simulink model "Mechanical_sol"  (R2018b)
settings: Solver=VariableStepAuto  StartTime=0.0  StopTime=60  RelTol=1e-3
values from neighbouring files (symbols this model uses):
  Dm = 0.0071    [QuanserData.m]
  Dp = 0.0071    [QuanserData.m]
  Dt = 0.158    [QuanserData.m]
  g = 9.81    [QuanserData.m]
  Jeq = Jm+Jh+Jp    (= 1.120304e-05)    [QuanserData.m]
  Jp = 2.15e-2    (= 0.0215)    [QuanserData.m]
  k1 = 1.2e-5    (= 1.2e-05)    [QuanserData.m]
  k2 = 3.54e-9    (= 3.54e-09)    [QuanserData.m]
  k3 = 0    [QuanserData.m]
  k4 = 6.23e-7    (= 6.23e-07)    [QuanserData.m]
  km = 0.042    [QuanserData.m]
  Lm = 1.16e-3    (= 0.00116)    [QuanserData.m]
  Mb = 1.15    [QuanserData.m]
  Rm = 8.4    [QuanserData.m]
settings Model: Creator=y.briere  LastModifiedBy=y.briere
settings DataIOCC: InitialState=[]  LoadInitialState=on

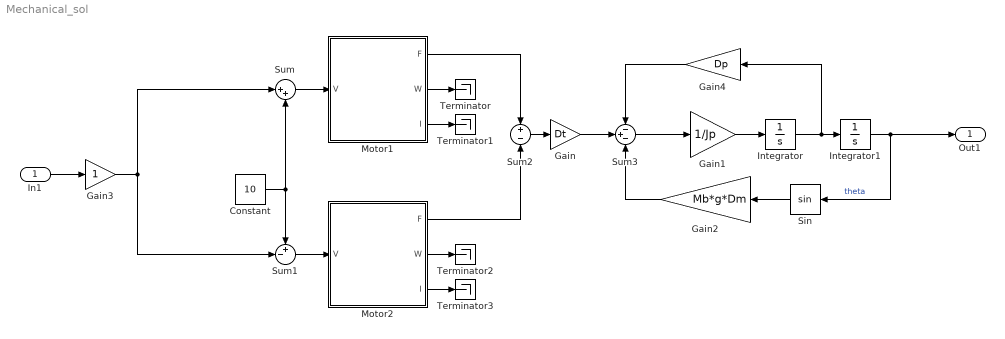
== system Mechanical_sol ==
  In1 : Inport
  Constant : Constant  Value=10
  Gain : Gain  Gain=Dt
  Gain1 : Gain  Gain=1/Jp
  Gain2 : Gain  Gain=Mb*g*Dm
  Gain3 : Gain
  Gain4 : Gain  Gain=Dp
  Integrator : Integrator
  Integrator1 : Integrator
  Motor1 : Subsystem
  Motor2 : Subsystem
  Sin : Trigonometry
  Sum : Sum  Inputs=|++
  Sum1 : Sum  Inputs=+-|
  Sum2 : Sum  Inputs=+-
  Sum3 : Sum  Inputs=-+-
  Terminator{,1..3} (4 alike) : Terminator
  Out1 : Outport
  wires:
  Sum1/1 -> Motor2/1(V)
  Sum/1 -> Motor1/1(V)
  Motor2/1(F) -> Sum2/2
  Motor1/1(F) -> Sum2/1
  Sum2/1 -> Gain/1
  Sum3/1 -> Gain1/1
  Integrator1/1 -> Sin/1, Out1/1  "theta"
  Gain1/1 -> Integrator/1
  Integrator/1 -> Gain4/1, Integrator1/1
  Sin/1 -> Gain2/1
  Motor1/2(W) -> Terminator/1
  Motor1/3(I) -> Terminator1/1
  Motor2/2(W) -> Terminator2/1
  Motor2/3(I) -> Terminator3/1
  Gain3/1 -> Sum/1, Sum1/2
  Constant/1 -> Sum/2, Sum1/1
  Gain4/1 -> Sum3/1
  Gain/1 -> Sum3/2
  Gain2/1 -> Sum3/3
  In1/1 -> Gain3/1

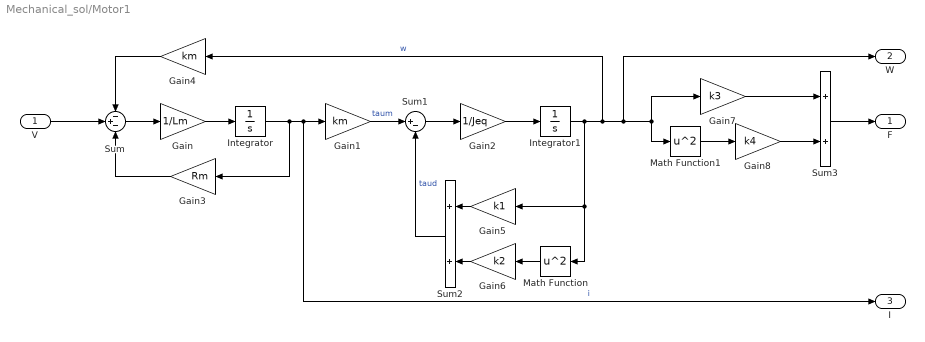
== system Mechanical_sol/Motor1 ==
  V : Inport
  Gain : Gain  Gain=1/Lm
  Gain1 : Gain  Gain=km
  Gain2 : Gain  Gain=1/Jeq
  Gain3 : Gain  Gain=Rm
  Gain4 : Gain  Gain=km
  Gain5 : Gain  Gain=k1
  Gain6 : Gain  Gain=k2
  Gain7 : Gain  Gain=k3
  Gain8 : Gain  Gain=k4
  Integrator : Integrator
  Integrator1 : Integrator
  Math Function : Math  Operator=square  SaturateOnIntegerOverflow=on
  Math Function1 : Math  Operator=square  SaturateOnIntegerOverflow=on
  Sum : Sum  Inputs=-+-
  Sum1 : Sum  Inputs=|+-
  Sum2 : Sum
  Sum3 : Sum
  F : Outport
  W : Outport  Port=2
  I : Outport  Port=3
  wires:
  Gain5/1 -> Sum2/1
  Sum3/1 -> F/1
  Gain8/1 -> Sum3/2
  Math Function/1 -> Gain6/1
  Gain4/1 -> Sum/1
  Gain/1 -> Integrator/1
  Math Function1/1 -> Gain8/1
  Sum1/1 -> Gain2/1
  Gain6/1 -> Sum2/2
  Sum2/1 -> Sum1/2  "taud"
  Integrator/1 -> I/1, Gain1/1, Gain3/1  "i"
  Sum/1 -> Gain/1
  Gain7/1 -> Sum3/1
  Integrator1/1 -> Gain5/1, Math Function/1, W/1, Gain7/1, Math Function1/1, Gain4/1  "w"
  Gain3/1 -> Sum/3
  Gain1/1 -> Sum1/1  "taum"
  Gain2/1 -> Integrator1/1
  V/1 -> Sum/2

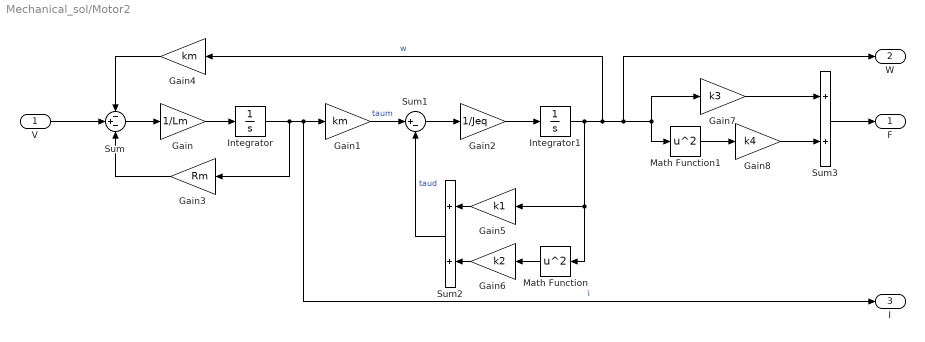
== system Mechanical_sol/Motor2 ==
  V : Inport
  Gain : Gain  Gain=1/Lm
  Gain1 : Gain  Gain=km
  Gain2 : Gain  Gain=1/Jeq
  Gain3 : Gain  Gain=Rm
  Gain4 : Gain  Gain=km
  Gain5 : Gain  Gain=k1
  Gain6 : Gain  Gain=k2
  Gain7 : Gain  Gain=k3
  Gain8 : Gain  Gain=k4
  Integrator : Integrator
  Integrator1 : Integrator
  Math Function : Math  Operator=square  SaturateOnIntegerOverflow=on
  Math Function1 : Math  Operator=square  SaturateOnIntegerOverflow=on
  Sum : Sum  Inputs=-+-
  Sum1 : Sum  Inputs=|+-
  Sum2 : Sum
  Sum3 : Sum
  F : Outport
  W : Outport  Port=2
  I : Outport  Port=3
  wires:
  V/1 -> Sum/2
  Gain2/1 -> Integrator1/1
  Gain1/1 -> Sum1/1  "taum"
  Gain3/1 -> Sum/3
  Integrator1/1 -> Gain4/1, Math Function1/1, Gain7/1, W/1, Math Function/1, Gain5/1  "w"
  Gain7/1 -> Sum3/1
  Sum/1 -> Gain/1
  Integrator/1 -> Gain3/1, Gain1/1, I/1  "i"
  Sum2/1 -> Sum1/2  "taud"
  Gain6/1 -> Sum2/2
  Sum1/1 -> Gain2/1
  Math Function1/1 -> Gain8/1
  Gain/1 -> Integrator/1
  Gain4/1 -> Sum/1
  Math Function/1 -> Gain6/1
  Gain8/1 -> Sum3/2
  Sum3/1 -> F/1
  Gain5/1 -> Sum2/1
